simulink model "Simulation_simulink_Mac"  (R2025b)
settings: Solver=FixedStepAuto  StartTime=0.0  StopTime=30  FixedStep=0.1  RelTol=1e-3  AbsTol=1e-3
StartFcn:
  | %Projet_SYS866_final;
values from neighbouring files (symbols this model uses):
  A_max = min(0.01 , A_min * factor)    [Projet_SYS866.m]    (also in Projet_SYS866_final.m; Simulation_matlab.m; Simulation_matlab_P2.m)
  A_min = coef * abs(dP_ref)^(n-0.5)    [Projet_SYS866.m]    (also in Projet_SYS866_final.m; Simulation_matlab.m; Simulation_matlab_P2.m)
  Kd = 0    [Projet_SYS866.m]    (also in Projet_SYS866_final.m)
  Ki = 0    [Projet_SYS866.m]    (also in Projet_SYS866_final.m = 0.04; Simulation_matlab.m = 0.04; Simulation_matlab_P2.m = 0.04)
  Kp = 2    [Projet_SYS866.m]    (also in Projet_SYS866_final.m = 0.4; Simulation_matlab.m = 0.4; Simulation_matlab_P2.m = 0.4)
  P_seuil = 0.5*Pc    (= 500)    [Projet_SYS866.m]    (also in Projet_SYS866_final.m; Simulation_matlab.m; Simulation_matlab_P2.m)
  Pc = 1000    [Projet_SYS866.m]    (also in Projet_SYS866_final.m; Simulation_matlab.m; Simulation_matlab_P2.m)
  Pc_ref = 1 / Pc    (= 0.001)    [Projet_SYS866_final.m]    (also in Simulation_matlab.m; Simulation_matlab_P2.m)
  rapport = A_min / A_max    [Projet_SYS866.m]    (also in Projet_SYS866_final.m; Simulation_matlab.m; Simulation_matlab_P2.m)
  saturation = 0.2    [Projet_SYS866_final.m]    (also in Simulation_matlab.m; Simulation_matlab_P2.m)
  tau_fan = mu_fan + sigma_fan*randn()    [Projet_SYS866.m]    (also in Projet_SYS866_final.m = 1; Simulation_matlab.m = 1; Simulation_matlab_P2.m = 1)
  Ts = 0.1    [Projet_SYS866.m]    (also in Projet_SYS866_final.m; Simulation_matlab.m; Simulation_matlab_P2.m)
  v_grow = max(0 , mu_v + sigma_v*randn())    [Projet_SYS866.m]    (also in Projet_SYS866_final.m; Simulation_matlab.m; Simulation_matlab_P2.m)
undefined symbols (not defined in the file or in its folder): DiscIntNeverNeededParam
libraries: fl_lib x4, nesl_utility x4, SimscapeFluids_lib x1, slpidlib x1
settings Model: PacingRate=0.900000  Creator=celin  LastModifiedBy=rmnlm
settings SolverCC: AutoScaleAbsTol=off  AlgebraicLoopSolver=TrustRegion  MaxZcPerStep=1.0
settings DebuggingCC: UnconnectedInputMsg=warning  UnconnectedOutputMsg=warning  UnconnectedLineMsg=warning  SymbolicDimsDataTypeCodeGenerationDiagnostic=none
settings ModelReferenceCC: EnableRefExpFcnMdlSchedulingChecks=on
settings SFSimCC: CustomCodeUndefinedFunction=UseInterfaceOnly
settings RTWCC: GPUComputeCapability=3.5  DLArmComputeVersion=19.05
settings SimscapeCC: SimscapeLogType=all  SimscapeLogSimulationStatistics=on  SimscapeLogDataHistory=10000.0

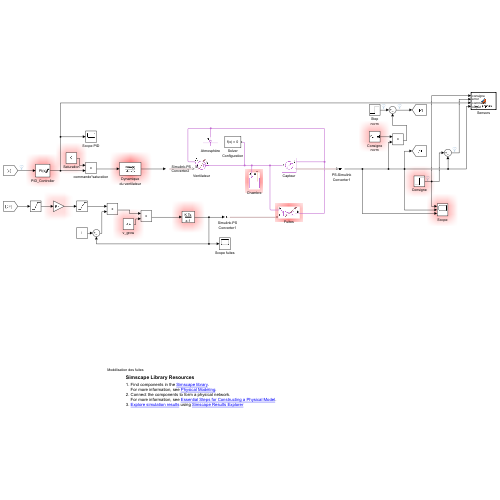
[thumbnail: Simulink's stored preview of the top-level diagram]
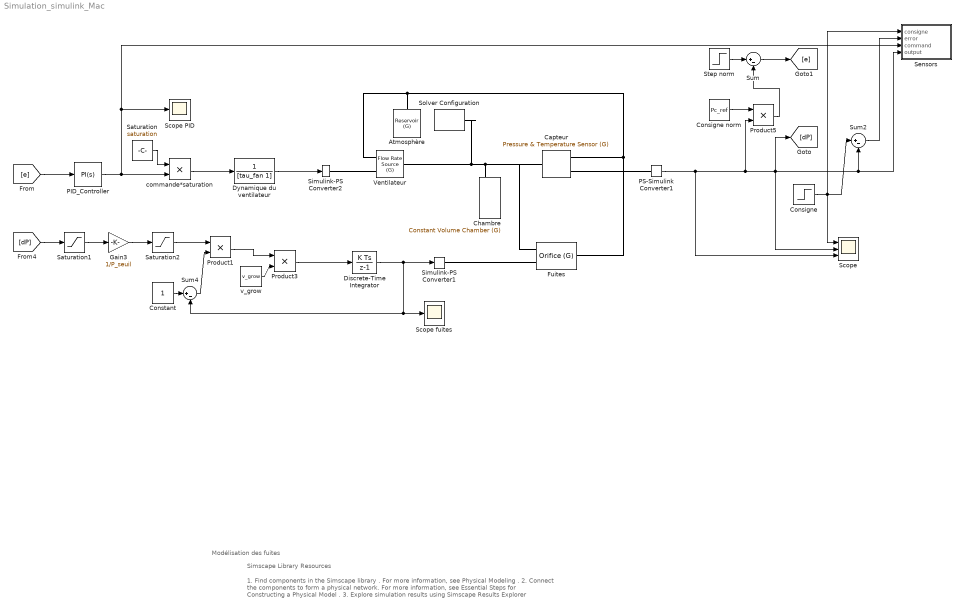
== system Simulation_simulink_Mac ==
  note: Modélisation des fuites
  note: 1. Find components in the Simscape library .
      | For more information, see Physical Modeling .
      | 2. Connect the components to form a physical network.
      | For more information, see Essential Steps for Constructing a Physical Model .
      | 3. Explore simulation results using Simscape Results Explorer
  note: Simscape Library Resources
  Atmosphère : fl_lib/Gas/Elements/Reservoir (G)  pressure_spec=foundation.enum.pressure_spec.atmospheric  reservoir_pressure=0.101325 MPa  reservoir_temperature=293.15 K  area_A=1 m^2
  Capteur : fl_lib/Gas/Sensors/Pressure & Temperature Sensor (G)  reference=foundation.enum.MeasurementReference.difference  pressure=true  pressure_spec=foundation.enum.PressureMeasementSpec.Absolute  temperature=false
      settings: InternalSimscapePortConfiguration="{\"Bottom\":[],\"Left\":[{\"id\":\"A\",\"label\":\"A\",\"type\":\"foundation.gas.gas\"}],\"Right\":[{\"id\":\"B\",\"label\":\"B\",\"type\":\"foundation.gas.gas\"},{\"id\":\"P\",\"label\":\"P\",\"type\":\"output\"}],\"Top\":[]}"
  Chambre : fl_lib/Gas/Elements/Constant Volume Chamber (G)  volume=V m^3  num_ports=foundation.enum.num_ports.one  area_A=0.1 m^2  area_B=0.01 m^2  area_C=0.01 m^2  area_D=0.01 m^2  p_I_specify=on  p_I_priority=High  p_I=0.101325 MPa  p_I_nominal_specify=on  p_I_nominal_value=1  p_I_nominal_unit=MPa  T_I_specify=off  T_I_priority=High  T_I=293.15 K  T_I_nominal_specify=off  T_I_nominal_value=1  T_I_nominal_unit=K  rho_I_specify=off  rho_I_priority=None  rho_I=1.2 kg/m^3  rho_I_nominal_specify=off  rho_I_nominal_value=1  rho_I_nominal_unit=kg/m^3
      settings: InternalSimscapePortConfiguration="{\"Bottom\":[],\"Left\":[{\"id\":\"A\",\"label\":\"A\",\"type\":\"foundation.gas.gas\"},{\"id\":\"H\",\"label\":\"H\",\"type\":\"foundation.thermal.thermal\"}],\"Right\":[],\"Top\":[]}"
  Consigne : Step  After=Pc  SampleTime=0
  Consigne norm : Constant  Value=Pc_ref
  Constant : Constant
  Discrete-Time Integrator : DiscreteIntegrator  gainval=1  InitialCondition=rapport  SampleTime=Ts  UpperSaturationLimit=A_max  LowerSaturationLimit=A_min  ICPrevOutput=DiscIntNeverNeededParam  ICPrevScaledInput=DiscIntNeverNeededParam
  Dynamique du ventilateur : TransferFcn  Denominator=[tau_fan 1]
  Fuites : SimscapeFluids_lib/Gas/Valves & Orifices/Orifice (G)  orifice_type=foundation.enum.constant_variable.variable  orifice_parameterization=fluids.gas.valves_orifices.enum.OrificeParameterization.Area  opening_characteristic=fluids.gas.valves_orifices.enum.OpeningCharacteristics.Linear  Cv_constant=4  Cv_max=4  L_Cv_TLU=0 : 0.2 : 1  Cv_TLU=[1e-06, .8, 1.6, 2.4, 3.2, 4]  xT_Cv=0.7  Kv_constant=3.6  Kv_max=K  L_Kv_TLU=0 : 0.2 : 1  Kv_TLU=[1e-06, .72, 1.44, 2.16, 2.88, 3.6]  xT_Kv=0.7  C_constant=12 l/(bar*s)  B_crit_constant=0.3  C_max=12 l/(bar*s)  B_crit_linear=0.3  L_C_TLU=0 : 0.2 : 1  C_TLU=[1e-05, 2.4, 4.8, 7.2, 9.6, 12] l/(bar*s)  B_crit_TLU=0.3 * ones(1, 6)  m=0.5  T_ref_C=293.15 K  rho_ref_C=1.185 kg/m^3  orifice_area_constant=1e-4 m^2  orifice_area_max=A_max m^2  L_orifice_area_TLU=0 : 0.2 : 1  orifice_area_TLU=[1e-10, 2e-05, 4e-05, 6e-05, 8e-05, .0001] m^2  Cd=0.64  leakage_fraction=1e-6  smoothing_factor=0.01  B_lam=0.999  area=10 m^2
      settings: InternalSimscapePortConfiguration="{\"Bottom\":[],\"Left\":[{\"id\":\"A\",\"label\":\"A\",\"type\":\"foundation.gas.gas\"},{\"id\":\"L\",\"label\":\"L\",\"type\":\"input\"}],\"Right\":[{\"id\":\"B\",\"label\":\"B\",\"type\":\"foundation.gas.gas\"}],\"Top\":[]}"
  Gain3 : Gain  Gain=1/P_seuil
  PID_Controller : slpidlib/PID Controller  Controller=PI  Form=Parallel  TimeDomain=Continuous-time  UseExternalTs=off  SampleTime=-1  IntegratorMethod=Forward Euler  FilterMethod=Forward Euler  ControllerParametersSource=internal  P=Kp  I=Ki  UseKiTs=off  D=Kd  UseExternalDerivativeSource=off  N=10  UseFilter=on  TunerSelectOption=Transfer Function Based (PID Tuner App)  InitialConditionSource=internal  InitialConditionForIntegrator=0  InitialConditionForFilter=0  DifferentiatorICPrevScaledInput=0  ExternalReset=none  TrackingMode=off  Kt=1  LimitOutput=on  SatLimitsSource=internal  UpperSaturationLimit=1  LowerSaturationLimit=0  LinearizeAsGain=off  AntiWindupMode=clamping  Kb=1  LimitIntegrator=off  UpperIntegratorSaturationLimit=1  LowerIntegratorSaturationLimit=-1  POutMin=[]  POutMax=[]  IOutMin=[]  IOutMax=[]  DOutMin=[]  DOutMax=[]  NOutMin=[]  NOutMax=[]  SumOutMin=[]  SumOutMax=[]  SaturationOutMin=[]  SaturationOutMax=[]  PParamMin=[]  PParamMax=[]  IParamMin=[]  IParamMax=[]  DParamMin=[]  DParamMax=[]  NParamMin=[]  NParamMax=[]  KbParamMin=[]  KbParamMax=[]  KtParamMin=[]  KtParamMax=[]  KbOutMin=[]  KbOutMax=[]  KtOutMin=[]  KtOutMax=[]  IntegratorOutMin=[]  IntegratorOutMax=[]  FilterOutMin=[]  FilterOutMax=[]  SumI1OutMin=[]  SumI1OutMax=[]  SumI2OutMin=[]  SumI2OutMax=[]  SumI3OutMin=[]  SumI3OutMax=[]  SumI4OutMin=[]  SumI4OutMax=[]  SumDOutMin=[]  SumDOutMax=[]  DifferentiatorOutMin=[]  DifferentiatorOutMax=[]  FilterDiffOutCoefMin=[]  FilterDiffOutCoefMax=[]  ReciprocalOutMin=[]  ReciprocalOutMax=[]  SumDenOutMin=[]  SumDenOutMax=[]  SumNumOutMin=[]  SumNumOutMax=[]  DivideOutMin=[]  DivideOutMax=[]  UdiffTsProdOutMin=[]  UdiffTsProdOutMax=[]  NTsProdOutMin=[]  NTsProdOutMax=[]  UintegralTsProdOutMin=[]  UintegralTsProdOutMax=[]  UngainTsProdOutMin=[]  UngainTsProdOutMax=[]  ClampingZeroOutDataTypeStr=Inherit: Inherit via back propagation  ClampingZeroOutMin=[]  ClampingZeroOutMax=[]  FilterDenConstantOutDataTypeStr=Inherit: Inherit via back propagation  FilterDenConstantOutMin=[]  FilterDenConstantOutMax=[]  PCopyOutDataTypeStr=Inherit: Inherit via back propagation  PCopyOutMin=[]  PCopyOutMax=[]  NCopyOutDataTypeStr=Inherit: Inherit via back propagation  NCopyOutMin=[]  NCopyOutMax=[]  IntegratorContinuousStateAttributes=''  IntegratorStateMustResolveToSignalObject=off  IntegratorRTWStateStorageClass=Auto  FilterContinuousStateAttributes=''  FilterStateMustResolveToSignalObject=off  FilterRTWStateStorageClass=Auto  ParallelPVariant=InternalParameters  IdealPVariant=Disabled  IVariant=InternalParameters  DVariant=Disabled  IntegratorVariant=Continuous  SatVariant=Enabled  AWVariant=ContClampingParallel  PCopyVariant=Disabled  TRVariant=Disabled  FdbkBlocksVariant=Forward  IdealPFdbkVariant=Disabled  SatFdbkVariant=Disabled  DerivativeFilterVariant=Disabled  NVariant=Disabled  NCopyVariant=Disabled_SignalSpec  FilterICVariant=Disabled  IntegratorICVariant=InternalICs  ExternalResetVariant=Disabled  TRSumVariant=Passthrough  SumFdbkVariant=Disabled  SumVariant=Sum_PI  TsampFilterVariant=InternalTs  TsampNgainVariant=Passthrough  TsampIntegralVariant=Disabled_SignalSpec  ExternalSaturationOutDataTypeStr=Inherit: Same as second input  DerivativeSourceVariant=Disabled  PreIntVariant=InternalPreInt
  PS-Simulink Converter1 : nesl_utility/PS-Simulink Converter  PhysicalDomain=network_engine_domain  SubClassName=ps_output  LeftPortType=input  RightPortType=output  PseudoPeriodic=off  Frequencies=[]  VectorFormat=inherit  Unit=inherit  AffineConversion=off
  Product1 : Product
  Product3 : Product
  Product5 : Product
  Saturation : Constant  Value=saturation
  Saturation1 : Saturate  UpperLimit=inf  LowerLimit=0
  Saturation2 : Saturate  UpperLimit=1  LowerLimit=0
  Scope : Scope  NumInputPorts=3
      settings: SampleTime=Ts  ActiveDisplayYMinimum=-163.18589559843196  ActiveDisplayYMaximum=1884.3969550577872
  Scope PID : Scope
      settings: ActiveDisplayYMinimum=-1.4877793943792328  ActiveDisplayYMaximum=1.6581154717107964
  Scope fuites : Scope
      settings: ActiveDisplayYMinimum=-0.049513946599008263  ActiveDisplayYMaximum=1.3843962287113007  DataLoggingVariableName=ScopeData2
  Sensors : MATLAB Function  TreatAsAtomicUnit=on
  Simulink-PS Converter1 : nesl_utility/Simulink-PS Converter  PhysicalDomain=network_engine_domain  SubClassName=ps_input  LeftPortType=input  RightPortType=output  PseudoPeriodic=off  Frequencies=[]  NoiseDistribution=none  NoiseParameters=[]  Unit=1  AffineConversion=off  FilteringAndDerivatives=provide  SimscapeFilterOrder=1  InputFilterTimeConstant=0.001  UdotUserProvided=0
  Simulink-PS Converter2 : nesl_utility/Simulink-PS Converter  PhysicalDomain=network_engine_domain  SubClassName=ps_input  LeftPortType=input  RightPortType=output  PseudoPeriodic=off  Frequencies=[]  NoiseDistribution=none  NoiseParameters=[]  Unit=1  AffineConversion=off  FilteringAndDerivatives=provide  SimscapeFilterOrder=1  InputFilterTimeConstant=0.001  UdotUserProvided=0
  Solver Configuration : nesl_utility/Solver Configuration  PhysicalDomain=network_engine_domain  SubClassName=solver  LeftPortType=input  RightPortType=generic  Tones=[]  Harmonics=[]  SimulateNoise=off  Profile=off  UseLocalSampling=off  EnableSwitchedLinearOptims=on  FrequencyDomain=off  UseCCode=off  RelTol=0.001  AbsTol=1e-06  MinStep=1e-09  ToWorkspace=off  RevertToSquareIcSolve=off  NumHomotopyIterations=100  PhasorMode=off  PhasorModeNumHarmonics=1  ConsistencySolver=NEWTON_XTOL_AFTER_FTOL  IndexReductionMethod=DerivativeReplacement  DoDC=off  ResidualTolerance=1e-09  ConsistencyTolSource=GLOBAL  ConsistencyAbsTol=0.001  ConsistencyRelTol=0.001  ConsistencyTolFactor=0.001  UseLocalSolver=off  LocalSolverChoice=NE_BACKWARD_EULER_ADVANCER  ResolveIndetEquations=on  FunctionEvalNumThread=1  LocalSolverSampleTime=0.001  DoFixedCost=off  MaxNonlinIter=3  MaxModeIter=2  ComputeImpulses=off  ImpulseIterations=2  LinearAlgebra=auto  LinearAlgebraNumThread=0  EquationFormulation=NE_TIME_EF  DelaysMemoryBudget=1024  AutomaticFiltering=on  FilteringTimeConstant=0.001  PartitionStorageMethod=AS_NEEDED  PartitionMemoryBudget=1024  PartitionMethod=ROBUST  MultibodyUseLocalSolver=off  MultibodyLocalSolverChoice=ODE1  MultibodyLocalSolverSampleTime=0.001
  Step norm : Step  SampleTime=0
  Sum : Sum  Inputs=|+-
  Sum2 : Sum  Inputs=|+-
  Sum4 : Sum  Inputs=|+-
  Ventilateur : fl_lib/Gas/Sources/Flow Rate Source (G)  source_type=foundation.enum.constant_controlled.controlled  flow_type=foundation.enum.mass_volumetric_flow.mass  mass_flow=0 kg/s  volumetric_flow=0 m^3/s  volumetric_flow_conditions=foundation.enum.volumetric_flow_conditions.actual  p_std=0.101325 MPa  T_std=20 degC  power_spec=foundation.enum.power_spec.isentropic  area_A=0.01 m^2  area_B=0.01 m^2
      settings: InternalSimscapePortConfiguration="{\"Bottom\":[],\"Left\":[{\"id\":\"A\",\"label\":\"A\",\"type\":\"foundation.gas.gas\"},{\"id\":\"M\",\"label\":\"M\",\"type\":\"input\"}],\"Right\":[{\"id\":\"B\",\"label\":\"B\",\"type\":\"foundation.gas.gas\"}],\"Top\":[]}"
  commande*saturation : Product
  v_grow : Constant  Value=v_grow
  wires:
  Step norm/1 -> Sum/1
  [e] -> PID_Controller/1
  PS-Simulink Converter1/1 -> Scope/2, [dP], Sum2/2, Sensors/4(output), Product5/2, Scope/3
  [dP] -> Saturation1/1
  Saturation1/1 -> Gain3/1
  Gain3/1 -> Saturation2/1
  Saturation2/1 -> Product1/1
  Product1/1 -> Product3/1
  v_grow/1 -> Product3/2
  Product3/1 -> Discrete-Time Integrator/1
  Sum/1 -> [e]
  Discrete-Time Integrator/1 -> Simulink-PS Converter1/1, Scope fuites/1, Sum4/2
  Consigne norm/1 -> Product5/1
  Product5/1 -> Sum/2
  Consigne/1 -> Sensors/1(consigne), Sum2/1, Scope/1
  commande*saturation/1 -> Dynamique du ventilateur/1
  Saturation/1 -> commande*saturation/1
  Constant/1 -> Sum4/1
  Sum4/1 -> Product1/2
  Dynamique du ventilateur/1 -> Simulink-PS Converter2/1
  PID_Controller/1 -> commande*saturation/2, Sensors/3(command), Scope PID/1
  Sum2/1 -> Sensors/2(error)
  connections:
  Simulink-PS Converter1/RConn1 -- Fuites/LConn2
  Solver Configuration/RConn1 -- Capteur/LConn1 -- Fuites/LConn1 -- Chambre/LConn1 -- Ventilateur/RConn1
  Simulink-PS Converter2/RConn1 -- Ventilateur/LConn2
  Fuites/RConn1 -- Ventilateur/LConn1 -- Atmosphère/LConn1 -- Capteur/RConn1
  Capteur/RConn2 -- PS-Simulink Converter1/LConn1

== matlab function Simulation_simulink_Mac/Sensors ==
  data: consigne input; error input; command input; output input
%MAC

function log_signals(consigne, error, command, output)
%#codegen

% Déclarer fopen/fprintf/fclose comme fonctions externes
coder.extrinsic('fopen','fprintf','fclose');

% Chemin du fichier CSV
filename = 'logs.csv';

% Ouvrir en mode append
fid = fopen(filename, 'a');

% Écrire une ligne CSV
fprintf(fid, '%f,%f,%f,%f\n', consigne, error, command, output);

% Fermer
fclose(fid);
end
